simulink library "TriphaseHardwaremodule"  (R2019b)
settings: Solver=ode45  StartTime=0.0  StopTime=10.0  RelTol=1e-3
values from neighbouring files (symbols this model uses):
  ControlSampleTime = 1/8000    (= 0.000125)    [initTPHardware.m]
  HWSampleTime = ControlSampleTime / Oversample    [Sim_TP3_VSM_init.m]    (also in initTPHardware.m = 3.125e-05)
  L1 = 0    [initVirtualCircuit.m]
undefined symbols (not defined in the file or in its folder): C1, C2, C_cap, C_CM, C_damp, C_DC, DT, gcbh, Iac_bit, Iac_max, L2, L_CM, LCL, PWM_f, R_C1, R_C2, R_cap, R_damp, R_L1, R_L2, sps_rtmsupport, Vac_bit, Vac_max, Vdc_bit, Vdc_max
libraries: $bdroot x58, powerlib x46, triphase_hpc x7, powerlib_meascontrol x5, simulink x2
(part 3 of 3)

== system TriphaseHardwaremodule/ctrlSelect4 ==
  ctrl : Inport
  Bus Creator{1..4} (4 alike) : BusCreator  Inputs=3
  Bus Selector : BusSelector  OutputSignals=pwm,connect,enable
  Data Type Conversion : DataTypeConversion  OutDataTypeStr=boolean
  Rate Transition : RateTransition  Integrity=off  Deterministic=off  OutPortSampleTime=0
  Selector1 : Selector  InputPortWidth=4  IndexOptions=Index vector (dialog)  Indices=[1]  OutputSizes=1
  Selector2 : Selector  InputPortWidth=4  IndexOptions=Index vector (dialog)  Indices=2  OutputSizes=1
  Selector3 : Selector  InputPortWidth=4  IndexOptions=Index vector (dialog)  Indices=3  OutputSizes=1
  Selector4 : Selector  InputPortWidth=4  IndexOptions=Index vector (dialog)  Indices=4  OutputSizes=1
  Sum of Elements : Sum  Inputs=+
  Sum of Elements1 : Sum  Inputs=+  SampleTime=ControlSampleTime
  ctrl1 : Outport  VectorParamsAs1DForOutWhenUnconnected=off
  ctrl2 : Outport  Port=2  VectorParamsAs1DForOutWhenUnconnected=off
  ctrl3 : Outport  Port=3  VectorParamsAs1DForOutWhenUnconnected=off
  ctrl4 : Outport  Port=4  VectorParamsAs1DForOutWhenUnconnected=off
  wires:
  Rate Transition/1 -> Selector1/1, Selector3/1, Selector4/1, Selector2/1
  Sum of Elements1/1 -> Data Type Conversion/1  "enable"
  Sum of Elements/1 -> Bus Creator4/2, Bus Creator2/2, Bus Creator3/2, Bus Creator1/2  "connect"
  Bus Creator4/1 -> ctrl4/1
  Selector4/1 -> Bus Creator4/1  "pwm"
  Bus Selector/1 -> Rate Transition/1  "<pwm>"
  Bus Selector/2 -> Sum of Elements/1  "<connect>"
  Selector1/1 -> Bus Creator1/1  "pwm"
  Bus Creator3/1 -> ctrl2/1
  Selector2/1 -> Bus Creator3/1  "pwm"
  Bus Creator1/1 -> ctrl1/1
  ctrl/1 -> Bus Selector/1
  Bus Selector/3 -> Sum of Elements1/1  "<enable>"
  Bus Creator2/1 -> ctrl3/1
  Selector3/1 -> Bus Creator2/1  "pwm"
  Data Type Conversion/1 -> Bus Creator4/3, Bus Creator2/3, Bus Creator3/3, Bus Creator1/3  "enable"

== system TriphaseHardwaremodule/emptyCtrl ==
  Bus Creator : BusCreator  Inputs=3
  Constant : Constant  Value=0
  Constant1 : Constant  Value=0
  Constant2 : Constant  Value=0
  ctrl : Outport  VectorParamsAs1DForOutWhenUnconnected=off
  wires:
  Constant1/1 -> Bus Creator/3  "enable"
  Bus Creator/1 -> ctrl/1
  Constant/1 -> Bus Creator/1  "pwm"
  Constant2/1 -> Bus Creator/2  "connect"

== system TriphaseHardwaremodule/emptyMeasure ==
  Bus Creator2 : BusCreator  Inputs=8
  Constant{,1..7} (8 alike) : Constant  Value=0
  meas : Outport  VectorParamsAs1DForOutWhenUnconnected=off
  wires:
  Constant4/1 -> Bus Creator2/6  "meas_i_out"
  Constant1/1 -> Bus Creator2/3  "meas_u_cap"
  Constant/1 -> Bus Creator2/1  "meas_u_dc"
  Bus Creator2/1 -> meas/1
  Constant2/1 -> Bus Creator2/4  "meas_u_out"
  Constant6/1 -> Bus Creator2/8  "enabled"
  Constant5/1 -> Bus Creator2/7  "connection_state"
  Constant3/1 -> Bus Creator2/5  "meas_i_inverter"
  Constant7/1 -> Bus Creator2/2  "meas_u_inverter"

== system TriphaseHardwaremodule/measMerge2 ==
  note: In Triphase Modell: Mittelwert aus allen dc Spannungen.
      | Da im Modell die DC Spannung identisch ist, wird die erste übergeben
  meas1 : Inport
  meas2 : Inport  Port=2
  Bus Creator2 : BusCreator  Inputs=8
  Bus Selector1 : BusSelector  OutputSignals=connection_state,enabled,meas_u_dc
  Bus Selector6 : BusSelector  OutputSignals=meas_u_inverter,meas_u_cap,meas_u_out,meas_i_inverter,meas_i_out
  Bus Selector7 : BusSelector  OutputSignals=meas_u_inverter,meas_u_cap,meas_u_out,meas_i_inverter,meas_i_out
  Mux{,1..4} (5 alike) : Mux  Inputs=2
  meas : Outport  VectorParamsAs1DForOutWhenUnconnected=off
  wires:
  Mux4/1 -> Bus Creator2/4  "meas_u_inverter"
  Bus Selector6/1 -> Mux4/1  "<meas_u_inverter>"
  Bus Selector7/1 -> Mux4/2  "<meas_u_inverter>"
  Bus Creator2/1 -> meas/1
  Bus Selector1/3 -> Bus Creator2/3  "<meas_u_dc>"
  Bus Selector1/2 -> Bus Creator2/2  "<enabled>"
  Bus Selector1/1 -> Bus Creator2/1  "<connection_state>"
  Bus Selector7/5 -> Mux3/2  "<meas_i_out>"
  Bus Selector6/5 -> Mux3/1  "<meas_i_out>"
  Bus Selector7/4 -> Mux2/2  "<meas_i_inverter>"
  Bus Selector6/4 -> Mux2/1  "<meas_i_inverter>"
  Bus Selector7/3 -> Mux1/2  "<meas_u_out>"
  Bus Selector6/3 -> Mux1/1  "<meas_u_out>"
  Bus Selector7/2 -> Mux/2  "<meas_u_cap>"
  Bus Selector6/2 -> Mux/1  "<meas_u_cap>"
  meas2/1 -> Bus Selector7/1  "meas2"
  meas1/1 -> Bus Selector6/1, Bus Selector1/1
  Mux/1 -> Bus Creator2/5  "meas_u_cap"
  Mux1/1 -> Bus Creator2/6  "meas_u_out"
  Mux2/1 -> Bus Creator2/7  "meas_i_inverter"
  Mux3/1 -> Bus Creator2/8  "meas_i_out"

== system TriphaseHardwaremodule/measMerge3 ==
  meas1 : Inport
  meas2 : Inport  Port=2
  meas3 : Inport  Port=3
  measMerge1 : $bdroot/measMerge2
  measMerge2 : $bdroot/measMerge2
  meas : Outport  VectorParamsAs1DForOutWhenUnconnected=off
  wires:
  meas1/1 -> measMerge2/1  "meas1"
  meas2/1 -> measMerge2/2  "meas2"
  measMerge2/1 -> measMerge1/1
  meas3/1 -> measMerge1/2  "meas3"
  measMerge1/1 -> meas/1

== system TriphaseHardwaremodule/measMerge4 ==
  note: In Triphase Modell: Mittelwert aus allen dc Spannungen.
      | Da im Modell die DC Spannung identisch ist, wird die erste übergeben
  meas1 : Inport
  meas2 : Inport  Port=2
  meas3 : Inport  Port=3
  meas4 : Inport  Port=4
  measMerge1 : $bdroot/measMerge2
  measMerge3 : $bdroot/measMerge3
  meas : Outport  VectorParamsAs1DForOutWhenUnconnected=off
  wires:
  meas1/1 -> measMerge3/1  "meas1"
  meas2/1 -> measMerge3/2  "meas2"
  meas3/1 -> measMerge3/3  "meas3"
  measMerge3/1 -> measMerge1/1
  meas4/1 -> measMerge1/2  "meas4"
  measMerge1/1 -> meas/1

== system TriphaseHardwaremodule/DC-Bus/ThreePhase IdealSwitch ==
  Gate : Inport
  Ideal Switch : powerlib/Power Electronics/Ideal Switch  Ron=0.001  Lon=0  IC=0  Rs=1e6  Cs=inf  Measurements=off
      settings: SourceProductName=Simscape Electrical
  Ideal Switch1 : powerlib/Power Electronics/Ideal Switch  Ron=0.001  Lon=0  IC=0  Rs=1e6  Cs=inf  Measurements=off
      settings: SourceProductName=Simscape Electrical
  Ideal Switch2 : powerlib/Power Electronics/Ideal Switch  Ron=0.001  Lon=0  IC=0  Rs=1e6  Cs=inf  Measurements=off
      settings: SourceProductName=Simscape Electrical
  a : PMIOPort  Side=Right
  A : PMIOPort  Port=2  Side=Left
  b : PMIOPort  Port=3  Side=Right
  B : PMIOPort  Port=4  Side=Left
  c : PMIOPort  Port=5  Side=Right
  C : PMIOPort  Port=6  Side=Left
  wires:
  Gate/1 -> Ideal Switch/1, Ideal Switch1/1, Ideal Switch2/1
  connections:
  Ideal Switch/RConn1 -- a/RConn1
  Ideal Switch1/RConn1 -- b/RConn1
  Ideal Switch/LConn1 -- A/RConn1
  Ideal Switch2/LConn1 -- C/RConn1
  Ideal Switch2/RConn1 -- c/RConn1
  Ideal Switch1/LConn1 -- B/RConn1

== system TriphaseHardwaremodule/Modul M30/B6 Brücke ==
  note: 1) Add Subsystem or Model blocks as valid variant choices.
      | 2) You cannot connect blocks at this level. At simulation, connectivity is automatically
      | determined, based on the active variant and port name matching.
  DutyCycle : Inport
  B6 Mittelwert : Subsystem  VariantControl=SimulationMode == 1
  B6 getaktet : Subsystem  VariantControl=SimulationMode == 2
  A : PMIOPort  Tag=PMCPort  Side=Left
  B : PMIOPort  Tag=PMCPort  Port=2  Side=Left
  C : PMIOPort  Tag=PMCPort  Port=3  Side=Left
  + : PMIOPort  Tag=PMCPort  Port=4  Side=Right
  - : PMIOPort  Tag=PMCPort  Port=5  Side=Right

== system TriphaseHardwaremodule/PWM delay AVG model4/Average ==
  In1 : Inport
  Enable : EnablePort
  Delay : Delay  DelayLength=round(ControlSampleTime/HWSampleTime/2)  InitialCondition=0
  Out1 : Outport  InitialOutput=0  VectorParamsAs1DForOutWhenUnconnected=off
  wires:
  In1/1 -> Delay/1
  Delay/1 -> Out1/1

== system TriphaseHardwaremodule/PWM delay AVG model4/Switched ==
  In1 : Inport
  Enable : EnablePort
  Out1 : Outport  InitialOutput=0  VectorParamsAs1DForOutWhenUnconnected=off
  wires:
  In1/1 -> Out1/1

== system TriphaseHardwaremodule/bridgefilter_1ph/B6 Brücke ==
  note: 1) Add Subsystem or Model blocks as valid variant choices.
      | 2) You cannot connect blocks at this level. At simulation, connectivity is automatically
      | determined, based on the active variant and port name matching.
  DutyCycle : Inport
  Enable : Inport  Port=2
  B6 Mittelwert : Subsystem  VariantControl=V_SIM_AVERAGE
  B6 getaktet : Subsystem  VariantControl=V_SIM_SWITCHED
  A : PMIOPort  Tag=PMCPort  Side=Left
  + : PMIOPort  Tag=PMCPort  Port=2  Side=Right
  - : PMIOPort  Tag=PMCPort  Port=3  Side=Right

== system TriphaseHardwaremodule/bridgefilter_1ph_PWMblock/B6 Brücke ==
  note: 1) Add Subsystem or Model blocks as valid variant choices.
      | 2) You cannot connect blocks at this level. At simulation, connectivity is automatically
      | determined, based on the active variant and port name matching.
  DutyCycle : Inport
  Enable : Inport  Port=2
  B6 Mittelwert : Subsystem  VariantControl=V_SIM_AVERAGE
  B6 getaktet : Subsystem  VariantControl=V_SIM_SWITCHED
  A : PMIOPort  Tag=PMCPort  Side=Left
  + : PMIOPort  Tag=PMCPort  Port=2  Side=Right
  - : PMIOPort  Tag=PMCPort  Port=3  Side=Right

== system TriphaseHardwaremodule/bridgefilter_1ph_PWMblock/PWM-Blocking ==
  "i_inv\t" : Inport
  Abs : Abs
  Compare To Constant1 : simulink/Logic and Bit Operations/Compare To Constant  relop=<=  const=I_BACK  OutDataTypeStr=boolean
  Compare To Constant2 : simulink/Logic and Bit Operations/Compare To Constant  relop=<=  const=I_MAX  OutDataTypeStr=boolean
  Switch : Switch  Criteria=u2 ~= 0
  Unit Delay : UnitDelay  InitialCondition=1  SampleTime=-1  HasFrameUpgradeWarning=on
  PWM_Ena : Outport  VectorParamsAs1DForOutWhenUnconnected=off
  wires:
  "i_inv\t"/1 -> Abs/1
  Abs/1 -> Compare To Constant2/1, Compare To Constant1/1
  Compare To Constant1/1 -> Switch/3
  Switch/1 -> PWM_Ena/1, Unit Delay/1
  Unit Delay/1 -> Switch/2
  Compare To Constant2/1 -> Switch/1

== system TriphaseHardwaremodule/Modul M30/B6 Brücke/B6 Mittelwert ==
  DutyCycle : Inport
  Universal Bridge : powerlib/Power Electronics/Universal Bridge  Arms=3  SnubberResistance=1e5  SnubberCapacitance=inf  Device=Average-model based VSC  Ron=1e-3  Lon=0  ForwardVoltages="[  0  0  ]"  ForwardVoltage=0  GTOparameters=[ 10e-6 , 20e-6 ]  IGBTparameters=[ 1e-6 , 2e-6 ]  Measurements=None  Measurements_2=None  converterType=Rectifier
      settings: SourceProductName=Simscape Electrical
  Universal Bridge1 : powerlib/Power Electronics/Universal Bridge  Arms=3  SnubberResistance=1e5  SnubberCapacitance=inf  Device=Diodes  Ron=1e-3  Lon=0  ForwardVoltages="[  0  0  ]"  ForwardVoltage=0  GTOparameters=[ 10e-6 , 20e-6 ]  IGBTparameters=[ 1e-6 , 2e-6 ]  Measurements=None  Measurements_2=None  converterType=Rectifier
      settings: SourceProductName=Simscape Electrical
  A : PMIOPort  Tag=PMCPort  Side=Left
  B : PMIOPort  Tag=PMCPort  Port=2  Side=Left
  C : PMIOPort  Tag=PMCPort  Port=3  Side=Left
  + : PMIOPort  Tag=PMCPort  Port=4  Side=Right
  - : PMIOPort  Tag=PMCPort  Port=5  Side=Right
  wires:
  DutyCycle/1 -> Universal Bridge/1
  connections:
  Universal Bridge1/LConn1 -- A/RConn1 -- Universal Bridge/LConn1
  Universal Bridge1/LConn2 -- B/RConn1 -- Universal Bridge/LConn2
  Universal Bridge1/LConn3 -- Universal Bridge/LConn3 -- C/RConn1
  Universal Bridge/RConn1 -- Universal Bridge1/RConn1 -- +/RConn1
  Universal Bridge/RConn2 -- -/RConn1 -- Universal Bridge1/RConn2

== system TriphaseHardwaremodule/Modul M30/B6 Brücke/B6 getaktet ==
  DutyCycle : Inport
  PWM Generator (2-Level) : powerlib_meascontrol/Pulse & Signal Generators/PWM Generator (2-Level)  ModulatorType=Three-phase bridge (6 pulses)  ModulatorMode=Unsynchronized  Fc=PWM_f  Pc=90  nF=27  MinMax="[ -1  1 ]"  SamplingTechnique=Natural  ModulatingSignals=off  m=0.8  Freq=60  Phase=0  Ts=0  ShowCarrierOutport=off
  Universal Bridge : powerlib/Power Electronics/Universal Bridge  Arms=3  SnubberResistance=1e5  SnubberCapacitance=inf  Device=IGBT / Diodes  Ron=1e-3  Lon=0  ForwardVoltages="[  0  0  ]"  ForwardVoltage=0  GTOparameters=[ 10e-6 , 20e-6 ]  IGBTparameters=[ DT , DT*2 ]  Measurements=None  Measurements_2=None  converterType=Rectifier
      settings: SourceProductName=Simscape Electrical
  A : PMIOPort  Tag=PMCPort  Side=Left
  B : PMIOPort  Tag=PMCPort  Port=2  Side=Left
  C : PMIOPort  Tag=PMCPort  Port=3  Side=Left
  + : PMIOPort  Tag=PMCPort  Port=4  Side=Right
  - : PMIOPort  Tag=PMCPort  Port=5  Side=Right
  wires:
  DutyCycle/1 -> PWM Generator (2-Level)/1
  PWM Generator (2-Level)/1 -> Universal Bridge/1
  connections:
  A/RConn1 -- Universal Bridge/LConn1
  B/RConn1 -- Universal Bridge/LConn2
  C/RConn1 -- Universal Bridge/LConn3
  -/RConn1 -- Universal Bridge/RConn2
  Universal Bridge/RConn1 -- +/RConn1

== system TriphaseHardwaremodule/bridgefilter_1ph/B6 Brücke/B6 Mittelwert ==
  DutyCycle : Inport
  Enable : Inport  Port=2
  Ideal Switch1 : powerlib/Power Electronics/Ideal Switch  Ron=0.001  Lon=0  IC=0  Rs=inf  Cs=inf  Measurements=off
      settings: SourceProductName=Simscape Electrical
  Product : Product
  Universal Bridge2 : powerlib/Power Electronics/Universal Bridge  Arms=1  SnubberResistance=1e5  SnubberCapacitance=inf  Device=Average-model based VSC  Ron=1e-3  Lon=0  ForwardVoltages="[  0  0  ]"  ForwardVoltage=0  GTOparameters=[ 10e-6 , 20e-6 ]  IGBTparameters=[ 1e-6 , 2e-6 ]  Measurements=None  Measurements_2=None  converterType=Rectifier
      settings: SourceProductName=Simscape Electrical
  Universal Bridge3 : powerlib/Power Electronics/Universal Bridge  Arms=1  SnubberResistance=1e5  SnubberCapacitance=inf  Device=Diodes  Ron=1e-3  Lon=0  ForwardVoltages="[  0  0  ]"  ForwardVoltage=0  GTOparameters=[ 10e-6 , 20e-6 ]  IGBTparameters=[ 1e-6 , 2e-6 ]  Measurements=None  Measurements_2=None  converterType=Rectifier
      settings: SourceProductName=Simscape Electrical
  A : PMIOPort  Tag=PMCPort  Side=Left
  + : PMIOPort  Tag=PMCPort  Port=2  Side=Right
  - : PMIOPort  Tag=PMCPort  Port=3  Side=Right
  wires:
  Enable/1 -> Ideal Switch1/1, Product/2
  DutyCycle/1 -> Product/1
  Product/1 -> Universal Bridge2/1
  connections:
  Universal Bridge2/RConn2 -- Universal Bridge3/RConn2 -- -/RConn1
  Universal Bridge2/RConn1 -- Universal Bridge3/RConn1 -- +/RConn1
  Universal Bridge3/LConn1 -- Ideal Switch1/LConn1 -- A/RConn1
  Ideal Switch1/RConn1 -- Universal Bridge2/LConn1

== system TriphaseHardwaremodule/bridgefilter_1ph/B6 Brücke/B6 getaktet ==
  DutyCycle : Inport
  Enable : Inport  Port=2
  On Delay : powerlib_meascontrol/Logic/On Delay  DelayType=On delay  delay=DT  ic=0  Ts=0
      settings: SourceProductName=Simscape Electrical
  PWM Generator (2-Level) : powerlib_meascontrol/Pulse & Signal Generators/PWM Generator (2-Level)  ModulatorType=Single-phase half-bridge (2 pulses)  ModulatorMode=Unsynchronized  Fc=PWM_f  Pc=0  nF=27  MinMax="[ -1  1 ]"  SamplingTechnique=Natural  ModulatingSignals=off  m=0.8  Freq=60  Phase=0  Ts=0  ShowCarrierOutport=off
  Product : Product
  Universal Bridge : powerlib/Power Electronics/Universal Bridge  Arms=1  SnubberResistance=1e5  SnubberCapacitance=inf  Device=MOSFET / Diodes  Ron=1e-3  Lon=0  ForwardVoltages="[  0  0  ]"  ForwardVoltage=0  GTOparameters=[ 10e-6 , 20e-6 ]  IGBTparameters=[ DT , DT*2 ]  Measurements=None  Measurements_2=None  converterType=Rectifier
      settings: SourceProductName=Simscape Electrical
  A : PMIOPort  Tag=PMCPort  Side=Left
  + : PMIOPort  Tag=PMCPort  Port=2  Side=Right
  - : PMIOPort  Tag=PMCPort  Port=3  Side=Right
  wires:
  DutyCycle/1 -> PWM Generator (2-Level)/1
  Product/1 -> Universal Bridge/1
  Enable/1 -> Product/2
  PWM Generator (2-Level)/1 -> On Delay/1
  On Delay/1 -> Product/1
  connections:
  A/RConn1 -- Universal Bridge/LConn1
  -/RConn1 -- Universal Bridge/RConn2
  Universal Bridge/RConn1 -- +/RConn1

== system TriphaseHardwaremodule/bridgefilter_1ph_PWMblock/B6 Brücke/B6 Mittelwert ==
  DutyCycle : Inport
  Enable : Inport  Port=2
  Ideal Switch1 : powerlib/Power Electronics/Ideal Switch  Ron=0.001  Lon=0  IC=0  Rs=inf  Cs=inf  Measurements=off
      settings: SourceProductName=Simscape Electrical
  Product : Product
  Universal Bridge2 : powerlib/Power Electronics/Universal Bridge  Arms=1  SnubberResistance=1e5  SnubberCapacitance=inf  Device=Average-model based VSC  Ron=1e-3  Lon=0  ForwardVoltages="[  0  0  ]"  ForwardVoltage=0  GTOparameters=[ 10e-6 , 20e-6 ]  IGBTparameters=[ 1e-6 , 2e-6 ]  Measurements=None  Measurements_2=None  converterType=Rectifier
      settings: SourceProductName=Simscape Electrical
  Universal Bridge3 : powerlib/Power Electronics/Universal Bridge  Arms=1  SnubberResistance=1e5  SnubberCapacitance=inf  Device=Diodes  Ron=1e-3  Lon=0  ForwardVoltages="[  0  0  ]"  ForwardVoltage=0  GTOparameters=[ 10e-6 , 20e-6 ]  IGBTparameters=[ 1e-6 , 2e-6 ]  Measurements=None  Measurements_2=None  converterType=Rectifier
      settings: SourceProductName=Simscape Electrical
  A : PMIOPort  Tag=PMCPort  Side=Left
  + : PMIOPort  Tag=PMCPort  Port=2  Side=Right
  - : PMIOPort  Tag=PMCPort  Port=3  Side=Right
  wires:
  Product/1 -> Universal Bridge2/1
  DutyCycle/1 -> Product/1
  Enable/1 -> Product/2, Ideal Switch1/1
  connections:
  Ideal Switch1/RConn1 -- Universal Bridge2/LConn1
  A/RConn1 -- Ideal Switch1/LConn1 -- Universal Bridge3/LConn1
  +/RConn1 -- Universal Bridge3/RConn1 -- Universal Bridge2/RConn1
  -/RConn1 -- Universal Bridge3/RConn2 -- Universal Bridge2/RConn2

== system TriphaseHardwaremodule/bridgefilter_1ph_PWMblock/B6 Brücke/B6 getaktet ==
  DutyCycle : Inport
  Enable : Inport  Port=2
  On Delay : powerlib_meascontrol/Logic/On Delay  DelayType=On delay  delay=DT  ic=0  Ts=0
      settings: SourceProductName=Simscape Electrical
  PWM Generator (2-Level) : powerlib_meascontrol/Pulse & Signal Generators/PWM Generator (2-Level)  ModulatorType=Single-phase half-bridge (2 pulses)  ModulatorMode=Unsynchronized  Fc=PWM_f  Pc=0  nF=27  MinMax="[ -1  1 ]"  SamplingTechnique=Natural  ModulatingSignals=off  m=0.8  Freq=60  Phase=0  Ts=0  ShowCarrierOutport=off
  Product : Product
  Universal Bridge : powerlib/Power Electronics/Universal Bridge  Arms=1  SnubberResistance=1e5  SnubberCapacitance=inf  Device=MOSFET / Diodes  Ron=1e-3  Lon=0  ForwardVoltages="[  0  0  ]"  ForwardVoltage=0  GTOparameters=[ 10e-6 , 20e-6 ]  IGBTparameters=[ DT , DT*2 ]  Measurements=None  Measurements_2=None  converterType=Rectifier
      settings: SourceProductName=Simscape Electrical
  A : PMIOPort  Tag=PMCPort  Side=Left
  + : PMIOPort  Tag=PMCPort  Port=2  Side=Right
  - : PMIOPort  Tag=PMCPort  Port=3  Side=Right
  wires:
  On Delay/1 -> Product/1
  PWM Generator (2-Level)/1 -> On Delay/1
  Enable/1 -> Product/2
  Product/1 -> Universal Bridge/1
  DutyCycle/1 -> PWM Generator (2-Level)/1
  connections:
  Universal Bridge/RConn1 -- +/RConn1
  -/RConn1 -- Universal Bridge/RConn2
  A/RConn1 -- Universal Bridge/LConn1
